simulink model "Approx_Multiplier_M3_AMA3"  (R2021a)
settings: Solver=VariableStepAuto  StartTime=0.0  StopTime=0.01  RelTol=1e-3
(part 1 of 3)
settings Model: SimulationMode=rapid-accelerator  Creator=PC  LastModifiedBy=chops

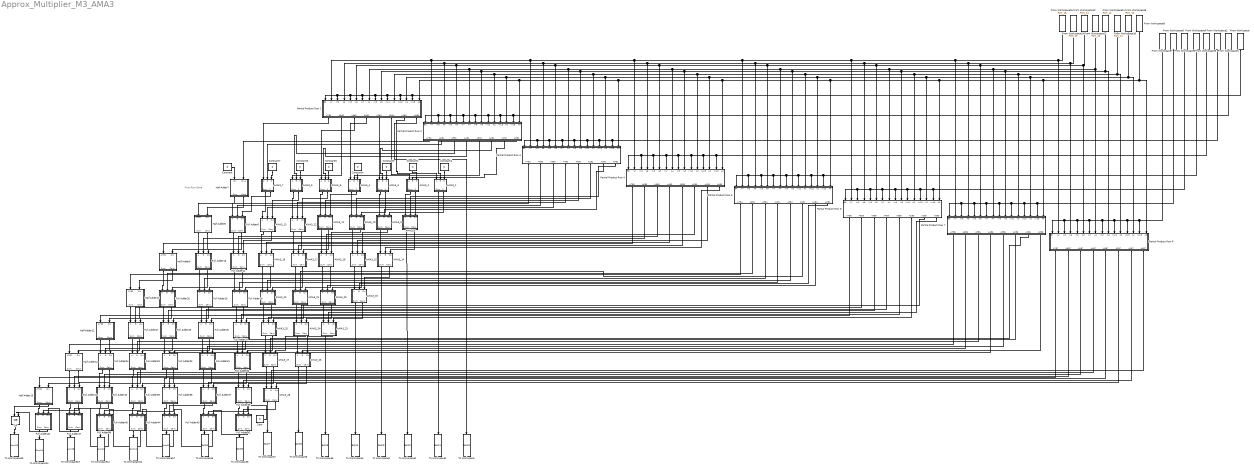
== system Approx_Multiplier_M3_AMA3 ==
  note: First Row Done
  AMA3_1 : Subsystem
  AMA3_10 : Subsystem
  AMA3_11 : Subsystem
  AMA3_12 : Subsystem
  AMA3_13 : Subsystem
  AMA3_14 : Subsystem
  AMA3_15 : Subsystem
  AMA3_16 : Subsystem
  AMA3_17 : Subsystem
  AMA3_18 : Subsystem
  AMA3_19 : Subsystem
  AMA3_2 : Subsystem
  AMA3_20 : Subsystem
  AMA3_21 : Subsystem
  AMA3_22 : Subsystem
  AMA3_23 : Subsystem
  AMA3_24 : Subsystem
  AMA3_25 : Subsystem
  AMA3_26 : Subsystem
  AMA3_27 : Subsystem
  AMA3_28 : Subsystem
  AMA3_3 : Subsystem
  AMA3_4 : Subsystem
  AMA3_5 : Subsystem
  AMA3_6 : Subsystem
  AMA3_7 : Subsystem
  AMA3_8 : Subsystem
  AMA3_9 : Subsystem
  Constant{,1..7} (8 alike) : Constant  Value=0
  From Workspace : FromWorkspace  VariableName=Port_1
  From Workspace1 : FromWorkspace  VariableName=Port_2
  From Workspace10 : FromWorkspace  VariableName=Port_11
  From Workspace11 : FromWorkspace  VariableName=Port_12
  From Workspace12 : FromWorkspace  VariableName=Port_13
  From Workspace13 : FromWorkspace  VariableName=Port_14
  From Workspace14 : FromWorkspace  VariableName=Port_15
  From Workspace15 : FromWorkspace  VariableName=Port_16
  From Workspace2 : FromWorkspace  VariableName=Port_3
  From Workspace3 : FromWorkspace  VariableName=Port_4
  From Workspace4 : FromWorkspace  VariableName=Port_5
  From Workspace5 : FromWorkspace  VariableName=Port_6
  From Workspace6 : FromWorkspace  VariableName=Port_7
  From Workspace7 : FromWorkspace  VariableName=Port_8
  From Workspace8 : FromWorkspace  VariableName=Port_9
  From Workspace9 : FromWorkspace  VariableName=Port_10
  Full Adder12 : Subsystem
  Full Adder13 : Subsystem
  Full Adder18 : Subsystem
  Full Adder19 : Subsystem
  Full Adder20 : Subsystem
  Full Adder24 : Subsystem
  Full Adder25 : Subsystem
  Full Adder26 : Subsystem
  Full Adder27 : Subsystem
  Full Adder30 : Subsystem
  Full Adder31 : Subsystem
  Full Adder32 : Subsystem
  Full Adder33 : Subsystem
  Full Adder34 : Subsystem
  Full Adder36 : Subsystem
  Full Adder37 : Subsystem
  Full Adder38 : Subsystem
  Full Adder39 : Subsystem
  Full Adder40 : Subsystem
  Full Adder41 : Subsystem
  Full Adder42 : Subsystem
  Full Adder43 : Subsystem
  Full Adder44 : Subsystem
  Full Adder45 : Subsystem
  Full Adder46 : Subsystem
  Full Adder47 : Subsystem
  Full Adder48 : Subsystem
  Full Adder6 : Subsystem
  Half Adder10 : Subsystem
  Half Adder11 : Subsystem
  Half Adder12 : Subsystem
  Half Adder13 : Subsystem
  Half Adder7 : Subsystem
  Half Adder8 : Subsystem
  Half Adder9 : Subsystem
  OR : Logic  Operator=OR  IconShape=distinctive  AllPortsSameDT=off  OutDataTypeStr=boolean
  Partial Product Row 1 : Subsystem
  Partial Product Row 2 : Subsystem
  Partial Product Row 3 : Subsystem
  Partial Product Row 4 : Subsystem
  Partial Product Row 5 : Subsystem
  Partial Product Row 6 : Subsystem
  Partial Product Row 7 : Subsystem
  Partial Product Row 8 : Subsystem
  To Workspace : ToWorkspace  VariableName=Sum0  SampleTime=0.01
      settings: Save2DSignal=2-D array (concatenate along first dimension)
  To Workspace1 : ToWorkspace  VariableName=Sum1  SampleTime=0.01
      settings: Save2DSignal=2-D array (concatenate along first dimension)
  To Workspace10 : ToWorkspace  VariableName=Sum10  SampleTime=0.01
      settings: Save2DSignal=2-D array (concatenate along first dimension)
  To Workspace11 : ToWorkspace  VariableName=Sum11  SampleTime=0.01
      settings: Save2DSignal=2-D array (concatenate along first dimension)
  To Workspace12 : ToWorkspace  VariableName=Sum12  SampleTime=0.01
      settings: Save2DSignal=2-D array (concatenate along first dimension)
  To Workspace13 : ToWorkspace  VariableName=Sum13  SampleTime=0.01
      settings: Save2DSignal=2-D array (concatenate along first dimension)
  To Workspace14 : ToWorkspace  VariableName=Sum14  SampleTime=0.01
      settings: Save2DSignal=2-D array (concatenate along first dimension)
  To Workspace15 : ToWorkspace  VariableName=Sum15  SampleTime=0.01
      settings: Save2DSignal=2-D array (concatenate along first dimension)
  To Workspace2 : ToWorkspace  VariableName=Sum2  SampleTime=0.01
      settings: Save2DSignal=2-D array (concatenate along first dimension)
  To Workspace3 : ToWorkspace  VariableName=Sum3  SampleTime=0.01
      settings: Save2DSignal=2-D array (concatenate along first dimension)
  To Workspace4 : ToWorkspace  VariableName=Sum4  SampleTime=0.01
      settings: Save2DSignal=2-D array (concatenate along first dimension)
  To Workspace5 : ToWorkspace  VariableName=Sum5  SampleTime=0.01
      settings: Save2DSignal=2-D array (concatenate along first dimension)
  To Workspace6 : ToWorkspace  VariableName=Sum6  SampleTime=0.01
      settings: Save2DSignal=2-D array (concatenate along first dimension)
  To Workspace7 : ToWorkspace  VariableName=Sum7  SampleTime=0.01
      settings: Save2DSignal=2-D array (concatenate along first dimension)
  To Workspace8 : ToWorkspace  VariableName=Sum8  SampleTime=0.01
      settings: Save2DSignal=2-D array (concatenate along first dimension)
  To Workspace9 : ToWorkspace  VariableName=Sum9  SampleTime=0.01
      settings: Save2DSignal=2-D array (concatenate along first dimension)
  Zero : Constant  Value=0  OutDataTypeStr=Inherit: Inherit via back propagation
  wires:
  Half Adder11/2(Cout) -> Half Adder12/2(Cin)
  AMA3_8/1(Sum) -> To Workspace2/1
  AMA3_12/2(Carry) -> AMA3_18/3(Cin)
  Full Adder46/1(Sum) -> To Workspace12/1
  Partial Product Row 1/5(A3B0) -> AMA3_3/1(A)
  Full Adder43/1(Sum) -> To Workspace9/1
  From Workspace13/1 -> Partial Product Row 8/6(A5), Partial Product Row 6/6(A5), Partial Product Row 3/6(A5), Partial Product Row 1/6(A5), Partial Product Row 2/6(A5), Partial Product Row 4/6(A5), Partial Product Row 5/6(A5), Partial Product Row 7/6(A5)
  AMA3_9/2(Carry) -> AMA3_15/3(Cin)
  Partial Product Row 2/5(A3B1) -> AMA3_4/2(B)
  Partial Product Row 7/2(A6B6) -> Full Adder34/2(B)
  Partial Product Row 1/4(A4B0) -> AMA3_4/1(A)
  Partial Product Row 8/6(A2B7) -> Full Adder37/2(B)
  Partial Product Row 8/3(A5B7) -> Full Adder40/2(B)
  AMA3_10/2(Carry) -> AMA3_16/3(Cin)
  Partial Product Row 6/8(A0B5) -> AMA3_23/2(B)
  AMA3_7/1(Sum) -> AMA3_13/1(A)
  Full Adder47/1(Sum) -> To Workspace13/1
  AMA3_9/1(Sum) -> AMA3_14/1(A)
  AMA3_5/1(Sum) -> AMA3_11/1(A)
  From Workspace7/1 -> Partial Product Row 8/11(In11), Partial Product Row 8/9(In9), Partial Product Row 8/7(In7), Partial Product Row 8/5(In5), Partial Product Row 8/3(In3), Partial Product Row 8/1(B7), Partial Product Row 8/13(In13), Partial Product Row 8/15(In15)
  AMA3_10/1(Sum) -> AMA3_15/1(A)
  Partial Product Row 4/6(A2B3) -> AMA3_16/2(B)
  Partial Product Row 3/5(A3B2) -> AMA3_11/2(B)
  Half Adder10/1(Sum) -> Full Adder27/1(A)
  AMA3_21/2(Carry) -> AMA3_25/3(Cin)
  Partial Product Row 1/8(A0B0) -> To Workspace/1
  AMA3_17/2(Carry) -> AMA3_22/3(Cin)
  Partial Product Row 7/8(A0B6) -> AMA3_26/2(B)
  Half Adder12/2(Cout) -> Half Adder13/2(Cin)
  AMA3_19/1(Sum) -> To Workspace4/1
  AMA3_21/1(Sum) -> AMA3_24/1(A)
  Full Adder43/2(Carry) -> Full Adder44/3(Cin)
  Full Adder20/2(Carry) -> Full Adder27/3(Cin)
  Partial Product Row 6/1(A7B5) -> Half Adder11/1(A7B2)
  Full Adder31/2(Carry) -> Full Adder38/3(Cin)
  Partial Product Row 3/3(A5B2) -> AMA3_13/2(B)
  From Workspace5/1 -> Partial Product Row 6/7(In7), Partial Product Row 6/5(In5), Partial Product Row 6/1(B5), Partial Product Row 6/3(In3), Partial Product Row 6/9(In9), Partial Product Row 6/11(In11), Partial Product Row 6/13(In13), Partial Product Row 6/15(In15)
  AMA3_23/1(Sum) -> To Workspace5/1
  Partial Product Row 3/6(A2B2) -> AMA3_10/2(B)
  AMA3_4/1(Sum) -> AMA3_10/1(A)
  From Workspace11/1 -> Partial Product Row 8/10(A3), Partial Product Row 6/10(A3), Partial Product Row 4/10(A3), Partial Product Row 3/10(A3), Partial Product Row 1/10(A3), Partial Product Row 2/10(A3), Partial Product Row 5/10(A3), Partial Product Row 7/10(A3)
  Full Adder26/2(Carry) -> Full Adder33/3(Cin)
  From Workspace15/1 -> Partial Product Row 7/2(A7), Partial Product Row 5/2(A7), Partial Product Row 3/2(A7), Partial Product Row 1/2(A7), Partial Product Row 2/2(A7), Partial Product Row 4/2(A7), Partial Product Row 6/2(A7), Partial Product Row 8/2(A7)
  Partial Product Row 7/4(A4B6) -> Full Adder32/2(B)
  Full Adder31/1(Sum) -> Full Adder37/1(A)
  Full Adder24/2(Carry) -> Full Adder31/3(Cin)
  Full Adder34/1(Sum) -> Full Adder40/1(A)
  Full Adder30/1(Sum) -> Full Adder36/1(A)
  Partial Product Row 6/2(A6B5) -> Full Adder27/2(B)
  Full Adder41/1(Sum) -> Full Adder47/1(A)
  Partial Product Row 2/2(A6B1) -> AMA3_7/2(B)
  Partial Product Row 8/7(A1B7) -> Full Adder36/2(B)
  From Workspace8/1 -> Partial Product Row 8/16(A0), Partial Product Row 7/16(A0), Partial Product Row 6/16(A0), Partial Product Row 4/16(A0), Partial Product Row 3/16(A0), Partial Product Row 1/16(A0), Partial Product Row 2/16(A0), Partial Product Row 5/16(A0)
  AMA3_15/1(Sum) -> AMA3_19/1(A)
  Half Adder7/1(Sum) -> Full Adder6/1(A)
  Constant/1 -> Half Adder7/1(Cin)
  AMA3_4/2(Carry) -> AMA3_11/3(Cin)
  AMA3_18/1(Sum) -> AMA3_22/1(A)
  Constant7/1 -> AMA3_7/3(Cin)
  Full Adder19/1(Sum) -> Full Adder25/1(A)
  Constant5/1 -> AMA3_5/3(Cin)
  AMA3_27/2(Carry) -> Full Adder36/3(Cin)
  Partial Product Row 6/3(A5B5) -> Full Adder26/2(B)
  Partial Product Row 2/1(A7B1) -> Half Adder7/2(Cin1)
  AMA3_2/1(Sum) -> AMA3_8/1(A)
  Partial Product Row 5/5(A3B4) -> AMA3_22/2(B)
  AMA3_20/2(Carry) -> AMA3_24/3(Cin)
  Partial Product Row 8/2(A6B7) -> Full Adder41/2(B)
  From Workspace2/1 -> Partial Product Row 3/13(In13), Partial Product Row 3/7(In7), Partial Product Row 3/5(In5), Partial Product Row 3/3(In3), Partial Product Row 3/1(B2), Partial Product Row 3/9(In9), Partial Product Row 3/11(In11), Partial Product Row 3/15(In15)
  Partial Product Row 2/8(A0B1) -> AMA3_1/2(B)
  Constant1/1 -> AMA3_1/3(Cin)
  Partial Product Row 3/4(A4B2) -> AMA3_12/2(B)
  Partial Product Row 5/2(A6B4) -> Full Adder20/2(B)
  Full Adder27/1(Sum) -> Full Adder33/1(A)
  AMA3_12/1(Sum) -> AMA3_17/1(A)
  AMA3_26/1(Sum) -> To Workspace6/1
  From Workspace10/1 -> Partial Product Row 8/12(A2), Partial Product Row 7/12(A2), Partial Product Row 5/12(A2), Partial Product Row 4/12(A2), Partial Product Row 3/12(A2), Partial Product Row 1/12(A2), Partial Product Row 2/12(A2), Partial Product Row 6/12(A2)
  Full Adder40/1(Sum) -> Full Adder46/1(A)
  Partial Product Row 6/5(A3B5) -> Full Adder24/2(B)
  AMA3_28/1(Sum) -> To Workspace7/1
  Partial Product Row 1/3(A5B0) -> AMA3_5/1(A)
  Constant6/1 -> AMA3_6/3(Cin)
  Half Adder8/1(Sum) -> Full Adder13/1(A)
  AMA3_17/1(Sum) -> AMA3_21/1(A)
  Partial Product Row 8/5(A3B7) -> Full Adder38/2(B)
  From Workspace1/1 -> Partial Product Row 2/15(In15), Partial Product Row 2/5(In5), Partial Product Row 2/3(In3), Partial Product Row 2/1(B1), Partial Product Row 2/7(In7), Partial Product Row 2/9(In9), Partial Product Row 2/11(In11), Partial Product Row 2/13(In13)
  AMA3_16/1(Sum) -> AMA3_20/1(A)
  Partial Product Row 7/1(A7B6) -> Half Adder12/1(A7B2)
  Partial Product Row 7/7(A1B6) -> AMA3_27/2(B)
  AMA3_15/2(Carry) -> AMA3_20/3(Cin)
  Partial Product Row 4/2(A6B3) -> Full Adder13/2(B)
  AMA3_2/2(Carry) -> AMA3_9/3(Cin)
  AMA3_3/1(Sum) -> AMA3_9/1(A)
  Full Adder42/2(Carry) -> Full Adder43/3(Cin)
  AMA3_24/2(Carry) -> AMA3_27/3(Cin)
  AMA3_13/1(Sum) -> AMA3_18/1(A)
  Full Adder32/1(Sum) -> Full Adder38/1(A)
  Full Adder37/1(Sum) -> Full Adder43/1(A)
  Partial Product Row 8/4(A4B7) -> Full Adder39/2(B)
  AMA3_1/1(Sum) -> To Workspace1/1
  AMA3_3/2(Carry) -> AMA3_10/3(Cin)
  Partial Product Row 1/6(A2B0) -> AMA3_2/1(A)
  Half Adder8/2(Cout) -> Half Adder9/2(Cin)
  Partial Product Row 4/4(A4B3) -> AMA3_18/2(B)
  Partial Product Row 6/6(A2B5) -> AMA3_25/2(B)
  Partial Product Row 5/3(A5B4) -> Full Adder19/2(B)
  From Workspace3/1 -> Partial Product Row 4/13(In13), Partial Product Row 4/11(In11), Partial Product Row 4/9(In9), Partial Product Row 4/5(In5), Partial Product Row 4/3(In3), Partial Product Row 4/1(B3), Partial Product Row 4/7(In7), Partial Product Row 4/15(In15)
  Full Adder12/2(Carry) -> Full Adder19/3(Cin)
  From Workspace6/1 -> Partial Product Row 7/13(In13), Partial Product Row 7/7(In7), Partial Product Row 7/5(In5), Partial Product Row 7/1(B6), Partial Product Row 7/3(In3), Partial Product Row 7/9(In9), Partial Product Row 7/11(In11), Partial Product Row 7/15(In15)
  Full Adder30/2(Carry) -> Full Adder37/3(Cin)
  AMA3_23/2(Carry) -> AMA3_26/3(Cin)
  Full Adder44/1(Sum) -> To Workspace10/1
  AMA3_6/2(Carry) -> AMA3_13/3(Cin)
  AMA3_16/2(Carry) -> AMA3_21/3(Cin)
  From Workspace14/1 -> Partial Product Row 8/4(A6), Partial Product Row 7/4(A6), Partial Product Row 6/4(A6), Partial Product Row 5/4(A6), Partial Product Row 4/4(A6), Partial Product Row 3/4(A6), Partial Product Row 1/4(A6), Partial Product Row 2/4(A6)
  Partial Product Row 5/7(A1B4) -> AMA3_20/2(B)
  Half Adder12/1(Sum) -> Full Adder41/1(A)
  Full Adder12/1(Sum) -> Full Adder18/1(A)
  Partial Product Row 4/1(A7B3) -> Half Adder9/1(A7B2)
  From Workspace4/1 -> Partial Product Row 5/15(In15), Partial Product Row 5/13(In13), Partial Product Row 5/11(In11), Partial Product Row 5/7(In7), Partial Product Row 5/5(In5), Partial Product Row 5/1(B4), Partial Product Row 5/3(In3), Partial Product Row 5/9(In9)
  Full Adder25/1(Sum) -> Full Adder31/1(A)
  AMA3_7/2(Carry) -> Full Adder6/3(Cin)
  Half Adder13/1(Sum) -> Full Adder48/1(A)
  Full Adder33/1(Sum) -> Full Adder39/1(A)
  From Workspace9/1 -> Partial Product Row 8/14(A1), Partial Product Row 7/14(A1), Partial Product Row 4/14(A1), Partial Product Row 1/14(A1), Partial Product Row 2/14(A1), Partial Product Row 3/14(A1), Partial Product Row 5/14(A1), Partial Product Row 6/14(A1)
  AMA3_14/1(Sum) -> To Workspace3/1
  AMA3_20/1(Sum) -> AMA3_23/1(A)
  Partial Product Row 1/1(A7B0) -> AMA3_7/1(A)
  Partial Product Row 7/3(A5B6) -> Full Adder33/2(B)
  Full Adder18/1(Sum) -> Full Adder24/1(A)
  From Workspace12/1 -> Partial Product Row 8/8(A4), Partial Product Row 6/8(A4), Partial Product Row 4/8(A4), Partial Product Row 3/8(A4), Partial Product Row 1/8(A4), Partial Product Row 2/8(A4), Partial Product Row 5/8(A4), Partial Product Row 7/8(A4)
  AMA3_11/2(Carry) -> AMA3_17/3(Cin)
  AMA3_19/2(Carry) -> AMA3_23/3(Cin)
  Full Adder26/1(Sum) -> Full Adder32/1(A)
  Partial Product Row 1/7(A1B0) -> AMA3_1/1(A)
  Full Adder46/2(Carry) -> Full Adder47/3(Cin)
  Partial Product Row 4/7(A1B3) -> AMA3_15/2(B)
  Partial Product Row 5/1(A7B4) -> Half Adder10/1(A7B2)
  Full Adder33/2(Carry) -> Full Adder40/3(Cin)
  Half Adder9/1(Sum) -> Full Adder20/1(A)
  Partial Product Row 4/3(A5B3) -> Full Adder12/2(B)
  Full Adder27/2(Carry) -> Full Adder34/3(Cin)
  Full Adder34/2(Carry) -> Full Adder41/3(Cin)
  Full Adder20/1(Sum) -> Full Adder26/1(A)
  Partial Product Row 8/8(A0B7) -> AMA3_28/2(B)
  AMA3_6/1(Sum) -> AMA3_12/1(A)
  Full Adder36/1(Sum) -> Full Adder42/1(A)
  Partial Product Row 2/7(A1B1) -> AMA3_2/2(B)
  Partial Product Row 5/6(A2B4) -> AMA3_21/2(B)
  Full Adder6/1(Sum) -> Full Adder12/1(A)
  Full Adder45/2(Carry) -> Full Adder46/3(Cin)
  AMA3_11/1(Sum) -> AMA3_16/1(A)
  AMA3_13/2(Carry) -> Full Adder12/3(Cin)
  Partial Product Row 2/4(A4B1) -> AMA3_5/2(B)
  Partial Product Row 4/8(A0B3) -> AMA3_14/2(B)
  Partial Product Row 2/3(A5B1) -> AMA3_6/2(B)
  Partial Product Row 6/4(A4B5) -> Full Adder25/2(B)
  AMA3_1/2(Carry) -> AMA3_8/3(Cin)
  Full Adder48/1(Sum) -> To Workspace14/1
  From Workspace/1 -> Partial Product Row 1/3(In3), Partial Product Row 1/1(B0), Partial Product Row 1/5(In5), Partial Product Row 1/7(In7), Partial Product Row 1/9(In9), Partial Product Row 1/11(In11), Partial Product Row 1/13(In13), Partial Product Row 1/15(In15)
  AMA3_8/2(Carry) -> AMA3_14/3(Cin)
  Half Adder10/2(Cout) -> Half Adder11/2(Cin)
  Partial Product Row 3/8(A0B2) -> AMA3_8/2(B)
  AMA3_18/2(Carry) -> Full Adder18/3(Cin)
  Full Adder13/2(Carry) -> Full Adder20/3(Cin)
  Partial Product Row 7/6(A2B6) -> Full Adder30/2(B)
  Constant3/1 -> AMA3_3/3(Cin)
  AMA3_27/1(Sum) -> AMA3_28/1(A)
  AMA3_25/2(Carry) -> Full Adder30/3(Cin)
  Full Adder25/2(Carry) -> Full Adder32/3(Cin)
  Partial Product Row 4/5(A3B3) -> AMA3_17/2(B)
  AMA3_25/1(Sum) -> AMA3_27/1(A)
  Full Adder42/1(Sum) -> To Workspace8/1
  Half Adder11/1(Sum) -> Full Adder34/1(A)
  AMA3_5/2(Carry) -> AMA3_12/3(Cin)
  Partial Product Row 6/7(A1B5) -> AMA3_24/2(B)
  Constant4/1 -> AMA3_4/3(Cin)
  Constant2/1 -> AMA3_2/3(Cin)
  Full Adder47/2(Carry) -> Full Adder48/3(Cin)
  Full Adder39/1(Sum) -> Full Adder45/1(A)
  Full Adder18/2(Carry) -> Full Adder25/3(Cin)
  Partial Product Row 7/5(A3B6) -> Full Adder31/2(B)
  Partial Product Row 5/4(A4B4) -> Full Adder18/2(B)
  Half Adder9/2(Cout) -> Half Adder10/2(Cin)
  Partial Product Row 3/1(A7B2) -> Half Adder8/1(A7B2)
  Half Adder7/2(Cout) -> Half Adder8/2(Cin)
  Partial Product Row 3/2(A6B2) -> Full Adder6/2(B)
  Partial Product Row 5/8(A0B4) -> AMA3_19/2(B)
  AMA3_22/1(Sum) -> AMA3_25/1(A)
  Partial Product Row 3/7(A1B2) -> AMA3_9/2(B)
  Full Adder44/2(Carry) -> Full Adder45/3(Cin)
  Partial Product Row 1/2(A6B0) -> AMA3_6/1(A)
  Partial Product Row 2/6(A2B1) -> AMA3_3/2(B)
  Full Adder6/2(Carry) -> Full Adder13/3(Cin)
  AMA3_14/2(Carry) -> AMA3_19/3(Cin)
  Partial Product Row 8/1(A7B7) -> Half Adder13/1(A7B2)
  Full Adder24/1(Sum) -> Full Adder30/1(A)
  Full Adder13/1(Sum) -> Full Adder19/1(A)
  Full Adder38/1(Sum) -> Full Adder44/1(A)
  Full Adder45/1(Sum) -> To Workspace11/1
  Full Adder32/2(Carry) -> Full Adder39/3(Cin)
  AMA3_22/2(Carry) -> Full Adder24/3(Cin)
  AMA3_24/1(Sum) -> AMA3_26/1(A)
  Full Adder19/2(Carry) -> Full Adder26/3(Cin)
  AMA3_26/2(Carry) -> AMA3_28/3(Cin)
  Full Adder48/2(Carry) -> OR/2
  Half Adder13/2(Cout) -> OR/1
  OR/1 -> To Workspace15/1
  AMA3_28/2(Carry) -> Full Adder42/2(B)
  Full Adder36/2(Carry) -> Full Adder43/2(B)
  Full Adder37/2(Carry) -> Full Adder44/2(B)
  Full Adder38/2(Carry) -> Full Adder45/2(B)
  Full Adder39/2(Carry) -> Full Adder46/2(B)
  Full Adder40/2(Carry) -> Full Adder47/2(B)
  Full Adder41/2(Carry) -> Full Adder48/2(B)
  Zero/1 -> Full Adder42/3(Cin)

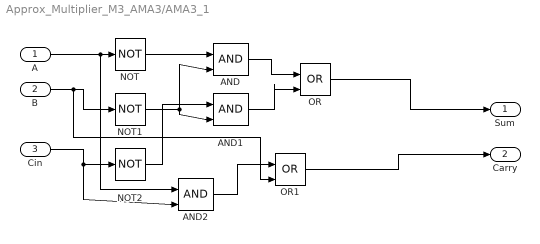
== system Approx_Multiplier_M3_AMA3/AMA3_1 ==
  A : Inport
  B : Inport  Port=2
  Cin : Inport  Port=3
  AND : Logic  IconShape=distinctive  AllPortsSameDT=off  OutDataTypeStr=boolean
  AND1 : Logic  IconShape=distinctive  AllPortsSameDT=off  OutDataTypeStr=boolean
  AND2 : Logic  IconShape=distinctive  AllPortsSameDT=off  OutDataTypeStr=boolean
  NOT : Logic  Operator=NOT  IconShape=distinctive  AllPortsSameDT=off  OutDataTypeStr=boolean
  NOT1 : Logic  Operator=NOT  IconShape=distinctive  AllPortsSameDT=off  OutDataTypeStr=boolean
  NOT2 : Logic  Operator=NOT  IconShape=distinctive  AllPortsSameDT=off  OutDataTypeStr=boolean
  OR : Logic  Operator=OR  IconShape=distinctive  AllPortsSameDT=off  OutDataTypeStr=boolean
  OR1 : Logic  Operator=OR  IconShape=distinctive  AllPortsSameDT=off  OutDataTypeStr=boolean
  Sum : Outport
  Carry : Outport  Port=2
  wires:
  A/1 -> AND2/1, NOT/1
  B/1 -> OR1/2, NOT1/1
  NOT/1 -> AND/1
  NOT1/1 -> AND1/2, AND/2
  Cin/1 -> AND2/2, NOT2/1
  NOT2/1 -> AND1/1
  AND/1 -> OR/1
  AND1/1 -> OR/2
  OR/1 -> Sum/1
  AND2/1 -> OR1/1
  OR1/1 -> Carry/1

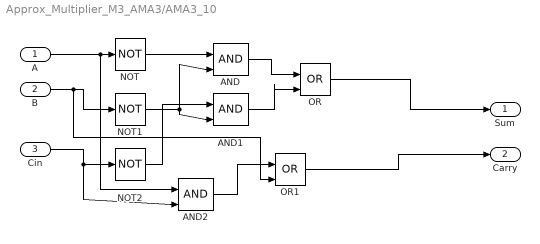
== system Approx_Multiplier_M3_AMA3/AMA3_10 ==
  A : Inport
  B : Inport  Port=2
  Cin : Inport  Port=3
  AND : Logic  IconShape=distinctive  AllPortsSameDT=off  OutDataTypeStr=boolean
  AND1 : Logic  IconShape=distinctive  AllPortsSameDT=off  OutDataTypeStr=boolean
  AND2 : Logic  IconShape=distinctive  AllPortsSameDT=off  OutDataTypeStr=boolean
  NOT : Logic  Operator=NOT  IconShape=distinctive  AllPortsSameDT=off  OutDataTypeStr=boolean
  NOT1 : Logic  Operator=NOT  IconShape=distinctive  AllPortsSameDT=off  OutDataTypeStr=boolean
  NOT2 : Logic  Operator=NOT  IconShape=distinctive  AllPortsSameDT=off  OutDataTypeStr=boolean
  OR : Logic  Operator=OR  IconShape=distinctive  AllPortsSameDT=off  OutDataTypeStr=boolean
  OR1 : Logic  Operator=OR  IconShape=distinctive  AllPortsSameDT=off  OutDataTypeStr=boolean
  Sum : Outport
  Carry : Outport  Port=2
  wires:
  A/1 -> AND2/1, NOT/1
  B/1 -> OR1/2, NOT1/1
  NOT/1 -> AND/1
  NOT1/1 -> AND1/2, AND/2
  Cin/1 -> AND2/2, NOT2/1
  NOT2/1 -> AND1/1
  AND/1 -> OR/1
  AND1/1 -> OR/2
  OR/1 -> Sum/1
  AND2/1 -> OR1/1
  OR1/1 -> Carry/1

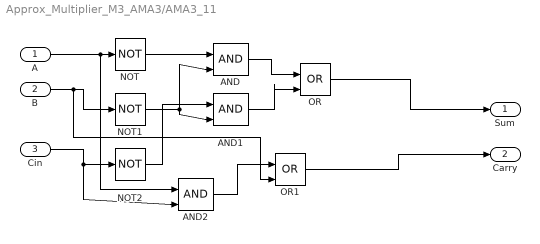
== system Approx_Multiplier_M3_AMA3/AMA3_11 ==
  A : Inport
  B : Inport  Port=2
  Cin : Inport  Port=3
  AND : Logic  IconShape=distinctive  AllPortsSameDT=off  OutDataTypeStr=boolean
  AND1 : Logic  IconShape=distinctive  AllPortsSameDT=off  OutDataTypeStr=boolean
  AND2 : Logic  IconShape=distinctive  AllPortsSameDT=off  OutDataTypeStr=boolean
  NOT : Logic  Operator=NOT  IconShape=distinctive  AllPortsSameDT=off  OutDataTypeStr=boolean
  NOT1 : Logic  Operator=NOT  IconShape=distinctive  AllPortsSameDT=off  OutDataTypeStr=boolean
  NOT2 : Logic  Operator=NOT  IconShape=distinctive  AllPortsSameDT=off  OutDataTypeStr=boolean
  OR : Logic  Operator=OR  IconShape=distinctive  AllPortsSameDT=off  OutDataTypeStr=boolean
  OR1 : Logic  Operator=OR  IconShape=distinctive  AllPortsSameDT=off  OutDataTypeStr=boolean
  Sum : Outport
  Carry : Outport  Port=2
  wires:
  A/1 -> AND2/1, NOT/1
  B/1 -> OR1/2, NOT1/1
  NOT/1 -> AND/1
  NOT1/1 -> AND1/2, AND/2
  Cin/1 -> AND2/2, NOT2/1
  NOT2/1 -> AND1/1
  AND/1 -> OR/1
  AND1/1 -> OR/2
  OR/1 -> Sum/1
  AND2/1 -> OR1/1
  OR1/1 -> Carry/1

== system Approx_Multiplier_M3_AMA3/AMA3_12 ==
  A : Inport
  B : Inport  Port=2
  Cin : Inport  Port=3
  AND : Logic  IconShape=distinctive  AllPortsSameDT=off  OutDataTypeStr=boolean
  AND1 : Logic  IconShape=distinctive  AllPortsSameDT=off  OutDataTypeStr=boolean
  AND2 : Logic  IconShape=distinctive  AllPortsSameDT=off  OutDataTypeStr=boolean
  NOT : Logic  Operator=NOT  IconShape=distinctive  AllPortsSameDT=off  OutDataTypeStr=boolean
  NOT1 : Logic  Operator=NOT  IconShape=distinctive  AllPortsSameDT=off  OutDataTypeStr=boolean
  NOT2 : Logic  Operator=NOT  IconShape=distinctive  AllPortsSameDT=off  OutDataTypeStr=boolean
  OR : Logic  Operator=OR  IconShape=distinctive  AllPortsSameDT=off  OutDataTypeStr=boolean
  OR1 : Logic  Operator=OR  IconShape=distinctive  AllPortsSameDT=off  OutDataTypeStr=boolean
  Sum : Outport
  Carry : Outport  Port=2
  wires:
  A/1 -> AND2/1, NOT/1
  B/1 -> OR1/2, NOT1/1
  NOT/1 -> AND/1
  NOT1/1 -> AND1/2, AND/2
  Cin/1 -> AND2/2, NOT2/1
  NOT2/1 -> AND1/1
  AND/1 -> OR/1
  AND1/1 -> OR/2
  OR/1 -> Sum/1
  AND2/1 -> OR1/1
  OR1/1 -> Carry/1

== system Approx_Multiplier_M3_AMA3/AMA3_13 ==
  A : Inport
  B : Inport  Port=2
  Cin : Inport  Port=3
  AND : Logic  IconShape=distinctive  AllPortsSameDT=off  OutDataTypeStr=boolean
  AND1 : Logic  IconShape=distinctive  AllPortsSameDT=off  OutDataTypeStr=boolean
  AND2 : Logic  IconShape=distinctive  AllPortsSameDT=off  OutDataTypeStr=boolean
  NOT : Logic  Operator=NOT  IconShape=distinctive  AllPortsSameDT=off  OutDataTypeStr=boolean
  NOT1 : Logic  Operator=NOT  IconShape=distinctive  AllPortsSameDT=off  OutDataTypeStr=boolean
  NOT2 : Logic  Operator=NOT  IconShape=distinctive  AllPortsSameDT=off  OutDataTypeStr=boolean
  OR : Logic  Operator=OR  IconShape=distinctive  AllPortsSameDT=off  OutDataTypeStr=boolean
  OR1 : Logic  Operator=OR  IconShape=distinctive  AllPortsSameDT=off  OutDataTypeStr=boolean
  Sum : Outport
  Carry : Outport  Port=2
  wires:
  A/1 -> AND2/1, NOT/1
  B/1 -> OR1/2, NOT1/1
  NOT/1 -> AND/1
  NOT1/1 -> AND1/2, AND/2
  Cin/1 -> AND2/2, NOT2/1
  NOT2/1 -> AND1/1
  AND/1 -> OR/1
  AND1/1 -> OR/2
  OR/1 -> Sum/1
  AND2/1 -> OR1/1
  OR1/1 -> Carry/1

== system Approx_Multiplier_M3_AMA3/AMA3_14 ==
  A : Inport
  B : Inport  Port=2
  Cin : Inport  Port=3
  AND : Logic  IconShape=distinctive  AllPortsSameDT=off  OutDataTypeStr=boolean
  AND1 : Logic  IconShape=distinctive  AllPortsSameDT=off  OutDataTypeStr=boolean
  AND2 : Logic  IconShape=distinctive  AllPortsSameDT=off  OutDataTypeStr=boolean
  NOT : Logic  Operator=NOT  IconShape=distinctive  AllPortsSameDT=off  OutDataTypeStr=boolean
  NOT1 : Logic  Operator=NOT  IconShape=distinctive  AllPortsSameDT=off  OutDataTypeStr=boolean
  NOT2 : Logic  Operator=NOT  IconShape=distinctive  AllPortsSameDT=off  OutDataTypeStr=boolean
  OR : Logic  Operator=OR  IconShape=distinctive  AllPortsSameDT=off  OutDataTypeStr=boolean
  OR1 : Logic  Operator=OR  IconShape=distinctive  AllPortsSameDT=off  OutDataTypeStr=boolean
  Sum : Outport
  Carry : Outport  Port=2
  wires:
  A/1 -> AND2/1, NOT/1
  B/1 -> OR1/2, NOT1/1
  NOT/1 -> AND/1
  NOT1/1 -> AND1/2, AND/2
  Cin/1 -> AND2/2, NOT2/1
  NOT2/1 -> AND1/1
  AND/1 -> OR/1
  AND1/1 -> OR/2
  OR/1 -> Sum/1
  AND2/1 -> OR1/1
  OR1/1 -> Carry/1

== system Approx_Multiplier_M3_AMA3/AMA3_15 ==
  A : Inport
  B : Inport  Port=2
  Cin : Inport  Port=3
  AND : Logic  IconShape=distinctive  AllPortsSameDT=off  OutDataTypeStr=boolean
  AND1 : Logic  IconShape=distinctive  AllPortsSameDT=off  OutDataTypeStr=boolean
  AND2 : Logic  IconShape=distinctive  AllPortsSameDT=off  OutDataTypeStr=boolean
  NOT : Logic  Operator=NOT  IconShape=distinctive  AllPortsSameDT=off  OutDataTypeStr=boolean
  NOT1 : Logic  Operator=NOT  IconShape=distinctive  AllPortsSameDT=off  OutDataTypeStr=boolean
  NOT2 : Logic  Operator=NOT  IconShape=distinctive  AllPortsSameDT=off  OutDataTypeStr=boolean
  OR : Logic  Operator=OR  IconShape=distinctive  AllPortsSameDT=off  OutDataTypeStr=boolean
  OR1 : Logic  Operator=OR  IconShape=distinctive  AllPortsSameDT=off  OutDataTypeStr=boolean
  Sum : Outport
  Carry : Outport  Port=2
  wires:
  A/1 -> AND2/1, NOT/1
  B/1 -> OR1/2, NOT1/1
  NOT/1 -> AND/1
  NOT1/1 -> AND1/2, AND/2
  Cin/1 -> AND2/2, NOT2/1
  NOT2/1 -> AND1/1
  AND/1 -> OR/1
  AND1/1 -> OR/2
  OR/1 -> Sum/1
  AND2/1 -> OR1/1
  OR1/1 -> Carry/1

== system Approx_Multiplier_M3_AMA3/AMA3_16 ==
  A : Inport
  B : Inport  Port=2
  Cin : Inport  Port=3
  AND : Logic  IconShape=distinctive  AllPortsSameDT=off  OutDataTypeStr=boolean
  AND1 : Logic  IconShape=distinctive  AllPortsSameDT=off  OutDataTypeStr=boolean
  AND2 : Logic  IconShape=distinctive  AllPortsSameDT=off  OutDataTypeStr=boolean
  NOT : Logic  Operator=NOT  IconShape=distinctive  AllPortsSameDT=off  OutDataTypeStr=boolean
  NOT1 : Logic  Operator=NOT  IconShape=distinctive  AllPortsSameDT=off  OutDataTypeStr=boolean
  NOT2 : Logic  Operator=NOT  IconShape=distinctive  AllPortsSameDT=off  OutDataTypeStr=boolean
  OR : Logic  Operator=OR  IconShape=distinctive  AllPortsSameDT=off  OutDataTypeStr=boolean
  OR1 : Logic  Operator=OR  IconShape=distinctive  AllPortsSameDT=off  OutDataTypeStr=boolean
  Sum : Outport
  Carry : Outport  Port=2
  wires:
  A/1 -> AND2/1, NOT/1
  B/1 -> OR1/2, NOT1/1
  NOT/1 -> AND/1
  NOT1/1 -> AND1/2, AND/2
  Cin/1 -> AND2/2, NOT2/1
  NOT2/1 -> AND1/1
  AND/1 -> OR/1
  AND1/1 -> OR/2
  OR/1 -> Sum/1
  AND2/1 -> OR1/1
  OR1/1 -> Carry/1

== system Approx_Multiplier_M3_AMA3/AMA3_17 ==
  A : Inport
  B : Inport  Port=2
  Cin : Inport  Port=3
  AND : Logic  IconShape=distinctive  AllPortsSameDT=off  OutDataTypeStr=boolean
  AND1 : Logic  IconShape=distinctive  AllPortsSameDT=off  OutDataTypeStr=boolean
  AND2 : Logic  IconShape=distinctive  AllPortsSameDT=off  OutDataTypeStr=boolean
  NOT : Logic  Operator=NOT  IconShape=distinctive  AllPortsSameDT=off  OutDataTypeStr=boolean
  NOT1 : Logic  Operator=NOT  IconShape=distinctive  AllPortsSameDT=off  OutDataTypeStr=boolean
  NOT2 : Logic  Operator=NOT  IconShape=distinctive  AllPortsSameDT=off  OutDataTypeStr=boolean
  OR : Logic  Operator=OR  IconShape=distinctive  AllPortsSameDT=off  OutDataTypeStr=boolean
  OR1 : Logic  Operator=OR  IconShape=distinctive  AllPortsSameDT=off  OutDataTypeStr=boolean
  Sum : Outport
  Carry : Outport  Port=2
  wires:
  A/1 -> AND2/1, NOT/1
  B/1 -> OR1/2, NOT1/1
  NOT/1 -> AND/1
  NOT1/1 -> AND1/2, AND/2
  Cin/1 -> AND2/2, NOT2/1
  NOT2/1 -> AND1/1
  AND/1 -> OR/1
  AND1/1 -> OR/2
  OR/1 -> Sum/1
  AND2/1 -> OR1/1
  OR1/1 -> Carry/1

== system Approx_Multiplier_M3_AMA3/AMA3_18 ==
  A : Inport
  B : Inport  Port=2
  Cin : Inport  Port=3
  AND : Logic  IconShape=distinctive  AllPortsSameDT=off  OutDataTypeStr=boolean
  AND1 : Logic  IconShape=distinctive  AllPortsSameDT=off  OutDataTypeStr=boolean
  AND2 : Logic  IconShape=distinctive  AllPortsSameDT=off  OutDataTypeStr=boolean
  NOT : Logic  Operator=NOT  IconShape=distinctive  AllPortsSameDT=off  OutDataTypeStr=boolean
  NOT1 : Logic  Operator=NOT  IconShape=distinctive  AllPortsSameDT=off  OutDataTypeStr=boolean
  NOT2 : Logic  Operator=NOT  IconShape=distinctive  AllPortsSameDT=off  OutDataTypeStr=boolean
  OR : Logic  Operator=OR  IconShape=distinctive  AllPortsSameDT=off  OutDataTypeStr=boolean
  OR1 : Logic  Operator=OR  IconShape=distinctive  AllPortsSameDT=off  OutDataTypeStr=boolean
  Sum : Outport
  Carry : Outport  Port=2
  wires:
  A/1 -> AND2/1, NOT/1
  B/1 -> OR1/2, NOT1/1
  NOT/1 -> AND/1
  NOT1/1 -> AND1/2, AND/2
  Cin/1 -> AND2/2, NOT2/1
  NOT2/1 -> AND1/1
  AND/1 -> OR/1
  AND1/1 -> OR/2
  OR/1 -> Sum/1
  AND2/1 -> OR1/1
  OR1/1 -> Carry/1

== system Approx_Multiplier_M3_AMA3/AMA3_19 ==
  A : Inport
  B : Inport  Port=2
  Cin : Inport  Port=3
  AND : Logic  IconShape=distinctive  AllPortsSameDT=off  OutDataTypeStr=boolean
  AND1 : Logic  IconShape=distinctive  AllPortsSameDT=off  OutDataTypeStr=boolean
  AND2 : Logic  IconShape=distinctive  AllPortsSameDT=off  OutDataTypeStr=boolean
  NOT : Logic  Operator=NOT  IconShape=distinctive  AllPortsSameDT=off  OutDataTypeStr=boolean
  NOT1 : Logic  Operator=NOT  IconShape=distinctive  AllPortsSameDT=off  OutDataTypeStr=boolean
  NOT2 : Logic  Operator=NOT  IconShape=distinctive  AllPortsSameDT=off  OutDataTypeStr=boolean
  OR : Logic  Operator=OR  IconShape=distinctive  AllPortsSameDT=off  OutDataTypeStr=boolean
  OR1 : Logic  Operator=OR  IconShape=distinctive  AllPortsSameDT=off  OutDataTypeStr=boolean
  Sum : Outport
  Carry : Outport  Port=2
  wires:
  A/1 -> AND2/1, NOT/1
  B/1 -> OR1/2, NOT1/1
  NOT/1 -> AND/1
  NOT1/1 -> AND1/2, AND/2
  Cin/1 -> AND2/2, NOT2/1
  NOT2/1 -> AND1/1
  AND/1 -> OR/1
  AND1/1 -> OR/2
  OR/1 -> Sum/1
  AND2/1 -> OR1/1
  OR1/1 -> Carry/1

== system Approx_Multiplier_M3_AMA3/AMA3_2 ==
  A : Inport
  B : Inport  Port=2
  Cin : Inport  Port=3
  AND : Logic  IconShape=distinctive  AllPortsSameDT=off  OutDataTypeStr=boolean
  AND1 : Logic  IconShape=distinctive  AllPortsSameDT=off  OutDataTypeStr=boolean
  AND2 : Logic  IconShape=distinctive  AllPortsSameDT=off  OutDataTypeStr=boolean
  NOT : Logic  Operator=NOT  IconShape=distinctive  AllPortsSameDT=off  OutDataTypeStr=boolean
  NOT1 : Logic  Operator=NOT  IconShape=distinctive  AllPortsSameDT=off  OutDataTypeStr=boolean
  NOT2 : Logic  Operator=NOT  IconShape=distinctive  AllPortsSameDT=off  OutDataTypeStr=boolean
  OR : Logic  Operator=OR  IconShape=distinctive  AllPortsSameDT=off  OutDataTypeStr=boolean
  OR1 : Logic  Operator=OR  IconShape=distinctive  AllPortsSameDT=off  OutDataTypeStr=boolean
  Sum : Outport
  Carry : Outport  Port=2
  wires:
  A/1 -> AND2/1, NOT/1
  B/1 -> OR1/2, NOT1/1
  NOT/1 -> AND/1
  NOT1/1 -> AND1/2, AND/2
  Cin/1 -> AND2/2, NOT2/1
  NOT2/1 -> AND1/1
  AND/1 -> OR/1
  AND1/1 -> OR/2
  OR/1 -> Sum/1
  AND2/1 -> OR1/1
  OR1/1 -> Carry/1

== system Approx_Multiplier_M3_AMA3/AMA3_20 ==
  A : Inport
  B : Inport  Port=2
  Cin : Inport  Port=3
  AND : Logic  IconShape=distinctive  AllPortsSameDT=off  OutDataTypeStr=boolean
  AND1 : Logic  IconShape=distinctive  AllPortsSameDT=off  OutDataTypeStr=boolean
  AND2 : Logic  IconShape=distinctive  AllPortsSameDT=off  OutDataTypeStr=boolean
  NOT : Logic  Operator=NOT  IconShape=distinctive  AllPortsSameDT=off  OutDataTypeStr=boolean
  NOT1 : Logic  Operator=NOT  IconShape=distinctive  AllPortsSameDT=off  OutDataTypeStr=boolean
  NOT2 : Logic  Operator=NOT  IconShape=distinctive  AllPortsSameDT=off  OutDataTypeStr=boolean
  OR : Logic  Operator=OR  IconShape=distinctive  AllPortsSameDT=off  OutDataTypeStr=boolean
  OR1 : Logic  Operator=OR  IconShape=distinctive  AllPortsSameDT=off  OutDataTypeStr=boolean
  Sum : Outport
  Carry : Outport  Port=2
  wires:
  A/1 -> AND2/1, NOT/1
  B/1 -> OR1/2, NOT1/1
  NOT/1 -> AND/1
  NOT1/1 -> AND1/2, AND/2
  Cin/1 -> AND2/2, NOT2/1
  NOT2/1 -> AND1/1
  AND/1 -> OR/1
  AND1/1 -> OR/2
  OR/1 -> Sum/1
  AND2/1 -> OR1/1
  OR1/1 -> Carry/1

== system Approx_Multiplier_M3_AMA3/AMA3_21 ==
  A : Inport
  B : Inport  Port=2
  Cin : Inport  Port=3
  AND : Logic  IconShape=distinctive  AllPortsSameDT=off  OutDataTypeStr=boolean
  AND1 : Logic  IconShape=distinctive  AllPortsSameDT=off  OutDataTypeStr=boolean
  AND2 : Logic  IconShape=distinctive  AllPortsSameDT=off  OutDataTypeStr=boolean
  NOT : Logic  Operator=NOT  IconShape=distinctive  AllPortsSameDT=off  OutDataTypeStr=boolean
  NOT1 : Logic  Operator=NOT  IconShape=distinctive  AllPortsSameDT=off  OutDataTypeStr=boolean
  NOT2 : Logic  Operator=NOT  IconShape=distinctive  AllPortsSameDT=off  OutDataTypeStr=boolean
  OR : Logic  Operator=OR  IconShape=distinctive  AllPortsSameDT=off  OutDataTypeStr=boolean
  OR1 : Logic  Operator=OR  IconShape=distinctive  AllPortsSameDT=off  OutDataTypeStr=boolean
  Sum : Outport
  Carry : Outport  Port=2
  wires:
  A/1 -> AND2/1, NOT/1
  B/1 -> OR1/2, NOT1/1
  NOT/1 -> AND/1
  NOT1/1 -> AND1/2, AND/2
  Cin/1 -> AND2/2, NOT2/1
  NOT2/1 -> AND1/1
  AND/1 -> OR/1
  AND1/1 -> OR/2
  OR/1 -> Sum/1
  AND2/1 -> OR1/1
  OR1/1 -> Carry/1

== system Approx_Multiplier_M3_AMA3/AMA3_22 ==
  A : Inport
  B : Inport  Port=2
  Cin : Inport  Port=3
  AND : Logic  IconShape=distinctive  AllPortsSameDT=off  OutDataTypeStr=boolean
  AND1 : Logic  IconShape=distinctive  AllPortsSameDT=off  OutDataTypeStr=boolean
  AND2 : Logic  IconShape=distinctive  AllPortsSameDT=off  OutDataTypeStr=boolean
  NOT : Logic  Operator=NOT  IconShape=distinctive  AllPortsSameDT=off  OutDataTypeStr=boolean
  NOT1 : Logic  Operator=NOT  IconShape=distinctive  AllPortsSameDT=off  OutDataTypeStr=boolean
  NOT2 : Logic  Operator=NOT  IconShape=distinctive  AllPortsSameDT=off  OutDataTypeStr=boolean
  OR : Logic  Operator=OR  IconShape=distinctive  AllPortsSameDT=off  OutDataTypeStr=boolean
  OR1 : Logic  Operator=OR  IconShape=distinctive  AllPortsSameDT=off  OutDataTypeStr=boolean
  Sum : Outport
  Carry : Outport  Port=2
  wires:
  A/1 -> AND2/1, NOT/1
  B/1 -> OR1/2, NOT1/1
  NOT/1 -> AND/1
  NOT1/1 -> AND1/2, AND/2
  Cin/1 -> AND2/2, NOT2/1
  NOT2/1 -> AND1/1
  AND/1 -> OR/1
  AND1/1 -> OR/2
  OR/1 -> Sum/1
  AND2/1 -> OR1/1
  OR1/1 -> Carry/1

== system Approx_Multiplier_M3_AMA3/AMA3_23 ==
  A : Inport
  B : Inport  Port=2
  Cin : Inport  Port=3
  AND : Logic  IconShape=distinctive  AllPortsSameDT=off  OutDataTypeStr=boolean
  AND1 : Logic  IconShape=distinctive  AllPortsSameDT=off  OutDataTypeStr=boolean
  AND2 : Logic  IconShape=distinctive  AllPortsSameDT=off  OutDataTypeStr=boolean
  NOT : Logic  Operator=NOT  IconShape=distinctive  AllPortsSameDT=off  OutDataTypeStr=boolean
  NOT1 : Logic  Operator=NOT  IconShape=distinctive  AllPortsSameDT=off  OutDataTypeStr=boolean
  NOT2 : Logic  Operator=NOT  IconShape=distinctive  AllPortsSameDT=off  OutDataTypeStr=boolean
  OR : Logic  Operator=OR  IconShape=distinctive  AllPortsSameDT=off  OutDataTypeStr=boolean
  OR1 : Logic  Operator=OR  IconShape=distinctive  AllPortsSameDT=off  OutDataTypeStr=boolean
  Sum : Outport
  Carry : Outport  Port=2
  wires:
  A/1 -> AND2/1, NOT/1
  B/1 -> OR1/2, NOT1/1
  NOT/1 -> AND/1
  NOT1/1 -> AND1/2, AND/2
  Cin/1 -> AND2/2, NOT2/1
  NOT2/1 -> AND1/1
  AND/1 -> OR/1
  AND1/1 -> OR/2
  OR/1 -> Sum/1
  AND2/1 -> OR1/1
  OR1/1 -> Carry/1

== system Approx_Multiplier_M3_AMA3/AMA3_24 ==
  A : Inport
  B : Inport  Port=2
  Cin : Inport  Port=3
  AND : Logic  IconShape=distinctive  AllPortsSameDT=off  OutDataTypeStr=boolean
  AND1 : Logic  IconShape=distinctive  AllPortsSameDT=off  OutDataTypeStr=boolean
  AND2 : Logic  IconShape=distinctive  AllPortsSameDT=off  OutDataTypeStr=boolean
  NOT : Logic  Operator=NOT  IconShape=distinctive  AllPortsSameDT=off  OutDataTypeStr=boolean
  NOT1 : Logic  Operator=NOT  IconShape=distinctive  AllPortsSameDT=off  OutDataTypeStr=boolean
  NOT2 : Logic  Operator=NOT  IconShape=distinctive  AllPortsSameDT=off  OutDataTypeStr=boolean
  OR : Logic  Operator=OR  IconShape=distinctive  AllPortsSameDT=off  OutDataTypeStr=boolean
  OR1 : Logic  Operator=OR  IconShape=distinctive  AllPortsSameDT=off  OutDataTypeStr=boolean
  Sum : Outport
  Carry : Outport  Port=2
  wires:
  A/1 -> AND2/1, NOT/1
  B/1 -> OR1/2, NOT1/1
  NOT/1 -> AND/1
  NOT1/1 -> AND1/2, AND/2
  Cin/1 -> AND2/2, NOT2/1
  NOT2/1 -> AND1/1
  AND/1 -> OR/1
  AND1/1 -> OR/2
  OR/1 -> Sum/1
  AND2/1 -> OR1/1
  OR1/1 -> Carry/1

== system Approx_Multiplier_M3_AMA3/AMA3_25 ==
  A : Inport
  B : Inport  Port=2
  Cin : Inport  Port=3
  AND : Logic  IconShape=distinctive  AllPortsSameDT=off  OutDataTypeStr=boolean
  AND1 : Logic  IconShape=distinctive  AllPortsSameDT=off  OutDataTypeStr=boolean
  AND2 : Logic  IconShape=distinctive  AllPortsSameDT=off  OutDataTypeStr=boolean
  NOT : Logic  Operator=NOT  IconShape=distinctive  AllPortsSameDT=off  OutDataTypeStr=boolean
  NOT1 : Logic  Operator=NOT  IconShape=distinctive  AllPortsSameDT=off  OutDataTypeStr=boolean
  NOT2 : Logic  Operator=NOT  IconShape=distinctive  AllPortsSameDT=off  OutDataTypeStr=boolean
  OR : Logic  Operator=OR  IconShape=distinctive  AllPortsSameDT=off  OutDataTypeStr=boolean
  OR1 : Logic  Operator=OR  IconShape=distinctive  AllPortsSameDT=off  OutDataTypeStr=boolean
  Sum : Outport
  Carry : Outport  Port=2
  wires:
  A/1 -> AND2/1, NOT/1
  B/1 -> OR1/2, NOT1/1
  NOT/1 -> AND/1
  NOT1/1 -> AND1/2, AND/2
  Cin/1 -> AND2/2, NOT2/1
  NOT2/1 -> AND1/1
  AND/1 -> OR/1
  AND1/1 -> OR/2
  OR/1 -> Sum/1
  AND2/1 -> OR1/1
  OR1/1 -> Carry/1

== system Approx_Multiplier_M3_AMA3/AMA3_26 ==
  A : Inport
  B : Inport  Port=2
  Cin : Inport  Port=3
  AND : Logic  IconShape=distinctive  AllPortsSameDT=off  OutDataTypeStr=boolean
  AND1 : Logic  IconShape=distinctive  AllPortsSameDT=off  OutDataTypeStr=boolean
  AND2 : Logic  IconShape=distinctive  AllPortsSameDT=off  OutDataTypeStr=boolean
  NOT : Logic  Operator=NOT  IconShape=distinctive  AllPortsSameDT=off  OutDataTypeStr=boolean
  NOT1 : Logic  Operator=NOT  IconShape=distinctive  AllPortsSameDT=off  OutDataTypeStr=boolean
  NOT2 : Logic  Operator=NOT  IconShape=distinctive  AllPortsSameDT=off  OutDataTypeStr=boolean
  OR : Logic  Operator=OR  IconShape=distinctive  AllPortsSameDT=off  OutDataTypeStr=boolean
  OR1 : Logic  Operator=OR  IconShape=distinctive  AllPortsSameDT=off  OutDataTypeStr=boolean
  Sum : Outport
  Carry : Outport  Port=2
  wires:
  A/1 -> AND2/1, NOT/1
  B/1 -> OR1/2, NOT1/1
  NOT/1 -> AND/1
  NOT1/1 -> AND1/2, AND/2
  Cin/1 -> AND2/2, NOT2/1
  NOT2/1 -> AND1/1
  AND/1 -> OR/1
  AND1/1 -> OR/2
  OR/1 -> Sum/1
  AND2/1 -> OR1/1
  OR1/1 -> Carry/1

== system Approx_Multiplier_M3_AMA3/AMA3_27 ==
  A : Inport
  B : Inport  Port=2
  Cin : Inport  Port=3
  AND : Logic  IconShape=distinctive  AllPortsSameDT=off  OutDataTypeStr=boolean
  AND1 : Logic  IconShape=distinctive  AllPortsSameDT=off  OutDataTypeStr=boolean
  AND2 : Logic  IconShape=distinctive  AllPortsSameDT=off  OutDataTypeStr=boolean
  NOT : Logic  Operator=NOT  IconShape=distinctive  AllPortsSameDT=off  OutDataTypeStr=boolean
  NOT1 : Logic  Operator=NOT  IconShape=distinctive  AllPortsSameDT=off  OutDataTypeStr=boolean
  NOT2 : Logic  Operator=NOT  IconShape=distinctive  AllPortsSameDT=off  OutDataTypeStr=boolean
  OR : Logic  Operator=OR  IconShape=distinctive  AllPortsSameDT=off  OutDataTypeStr=boolean
  OR1 : Logic  Operator=OR  IconShape=distinctive  AllPortsSameDT=off  OutDataTypeStr=boolean
  Sum : Outport
  Carry : Outport  Port=2
  wires:
  A/1 -> AND2/1, NOT/1
  B/1 -> OR1/2, NOT1/1
  NOT/1 -> AND/1
  NOT1/1 -> AND1/2, AND/2
  Cin/1 -> AND2/2, NOT2/1
  NOT2/1 -> AND1/1
  AND/1 -> OR/1
  AND1/1 -> OR/2
  OR/1 -> Sum/1
  AND2/1 -> OR1/1
  OR1/1 -> Carry/1

== system Approx_Multiplier_M3_AMA3/AMA3_28 ==
  A : Inport
  B : Inport  Port=2
  Cin : Inport  Port=3
  AND : Logic  IconShape=distinctive  AllPortsSameDT=off  OutDataTypeStr=boolean
  AND1 : Logic  IconShape=distinctive  AllPortsSameDT=off  OutDataTypeStr=boolean
  AND2 : Logic  IconShape=distinctive  AllPortsSameDT=off  OutDataTypeStr=boolean
  NOT : Logic  Operator=NOT  IconShape=distinctive  AllPortsSameDT=off  OutDataTypeStr=boolean
  NOT1 : Logic  Operator=NOT  IconShape=distinctive  AllPortsSameDT=off  OutDataTypeStr=boolean
  NOT2 : Logic  Operator=NOT  IconShape=distinctive  AllPortsSameDT=off  OutDataTypeStr=boolean
  OR : Logic  Operator=OR  IconShape=distinctive  AllPortsSameDT=off  OutDataTypeStr=boolean
  OR1 : Logic  Operator=OR  IconShape=distinctive  AllPortsSameDT=off  OutDataTypeStr=boolean
  Sum : Outport
  Carry : Outport  Port=2
  wires:
  A/1 -> AND2/1, NOT/1
  B/1 -> OR1/2, NOT1/1
  NOT/1 -> AND/1
  NOT1/1 -> AND1/2, AND/2
  Cin/1 -> AND2/2, NOT2/1
  NOT2/1 -> AND1/1
  AND/1 -> OR/1
  AND1/1 -> OR/2
  OR/1 -> Sum/1
  AND2/1 -> OR1/1
  OR1/1 -> Carry/1

== system Approx_Multiplier_M3_AMA3/AMA3_3 ==
  A : Inport
  B : Inport  Port=2
  Cin : Inport  Port=3
  AND : Logic  IconShape=distinctive  AllPortsSameDT=off  OutDataTypeStr=boolean
  AND1 : Logic  IconShape=distinctive  AllPortsSameDT=off  OutDataTypeStr=boolean
  AND2 : Logic  IconShape=distinctive  AllPortsSameDT=off  OutDataTypeStr=boolean
  NOT : Logic  Operator=NOT  IconShape=distinctive  AllPortsSameDT=off  OutDataTypeStr=boolean
  NOT1 : Logic  Operator=NOT  IconShape=distinctive  AllPortsSameDT=off  OutDataTypeStr=boolean
  NOT2 : Logic  Operator=NOT  IconShape=distinctive  AllPortsSameDT=off  OutDataTypeStr=boolean
  OR : Logic  Operator=OR  IconShape=distinctive  AllPortsSameDT=off  OutDataTypeStr=boolean
  OR1 : Logic  Operator=OR  IconShape=distinctive  AllPortsSameDT=off  OutDataTypeStr=boolean
  Sum : Outport
  Carry : Outport  Port=2
  wires:
  A/1 -> AND2/1, NOT/1
  B/1 -> OR1/2, NOT1/1
  NOT/1 -> AND/1
  NOT1/1 -> AND1/2, AND/2
  Cin/1 -> AND2/2, NOT2/1
  NOT2/1 -> AND1/1
  AND/1 -> OR/1
  AND1/1 -> OR/2
  OR/1 -> Sum/1
  AND2/1 -> OR1/1
  OR1/1 -> Carry/1

== system Approx_Multiplier_M3_AMA3/AMA3_4 ==
  A : Inport
  B : Inport  Port=2
  Cin : Inport  Port=3
  AND : Logic  IconShape=distinctive  AllPortsSameDT=off  OutDataTypeStr=boolean
  AND1 : Logic  IconShape=distinctive  AllPortsSameDT=off  OutDataTypeStr=boolean
  AND2 : Logic  IconShape=distinctive  AllPortsSameDT=off  OutDataTypeStr=boolean
  NOT : Logic  Operator=NOT  IconShape=distinctive  AllPortsSameDT=off  OutDataTypeStr=boolean
  NOT1 : Logic  Operator=NOT  IconShape=distinctive  AllPortsSameDT=off  OutDataTypeStr=boolean
  NOT2 : Logic  Operator=NOT  IconShape=distinctive  AllPortsSameDT=off  OutDataTypeStr=boolean
  OR : Logic  Operator=OR  IconShape=distinctive  AllPortsSameDT=off  OutDataTypeStr=boolean
  OR1 : Logic  Operator=OR  IconShape=distinctive  AllPortsSameDT=off  OutDataTypeStr=boolean
  Sum : Outport
  Carry : Outport  Port=2
  wires:
  A/1 -> AND2/1, NOT/1
  B/1 -> OR1/2, NOT1/1
  NOT/1 -> AND/1
  NOT1/1 -> AND1/2, AND/2
  Cin/1 -> AND2/2, NOT2/1
  NOT2/1 -> AND1/1
  AND/1 -> OR/1
  AND1/1 -> OR/2
  OR/1 -> Sum/1
  AND2/1 -> OR1/1
  OR1/1 -> Carry/1

== system Approx_Multiplier_M3_AMA3/AMA3_5 ==
  A : Inport
  B : Inport  Port=2
  Cin : Inport  Port=3
  AND : Logic  IconShape=distinctive  AllPortsSameDT=off  OutDataTypeStr=boolean
  AND1 : Logic  IconShape=distinctive  AllPortsSameDT=off  OutDataTypeStr=boolean
  AND2 : Logic  IconShape=distinctive  AllPortsSameDT=off  OutDataTypeStr=boolean
  NOT : Logic  Operator=NOT  IconShape=distinctive  AllPortsSameDT=off  OutDataTypeStr=boolean
  NOT1 : Logic  Operator=NOT  IconShape=distinctive  AllPortsSameDT=off  OutDataTypeStr=boolean
  NOT2 : Logic  Operator=NOT  IconShape=distinctive  AllPortsSameDT=off  OutDataTypeStr=boolean
  OR : Logic  Operator=OR  IconShape=distinctive  AllPortsSameDT=off  OutDataTypeStr=boolean
  OR1 : Logic  Operator=OR  IconShape=distinctive  AllPortsSameDT=off  OutDataTypeStr=boolean
  Sum : Outport
  Carry : Outport  Port=2
  wires:
  A/1 -> AND2/1, NOT/1
  B/1 -> OR1/2, NOT1/1
  NOT/1 -> AND/1
  NOT1/1 -> AND1/2, AND/2
  Cin/1 -> AND2/2, NOT2/1
  NOT2/1 -> AND1/1
  AND/1 -> OR/1
  AND1/1 -> OR/2
  OR/1 -> Sum/1
  AND2/1 -> OR1/1
  OR1/1 -> Carry/1

== system Approx_Multiplier_M3_AMA3/AMA3_6 ==
  A : Inport
  B : Inport  Port=2
  Cin : Inport  Port=3
  AND : Logic  IconShape=distinctive  AllPortsSameDT=off  OutDataTypeStr=boolean
  AND1 : Logic  IconShape=distinctive  AllPortsSameDT=off  OutDataTypeStr=boolean
  AND2 : Logic  IconShape=distinctive  AllPortsSameDT=off  OutDataTypeStr=boolean
  NOT : Logic  Operator=NOT  IconShape=distinctive  AllPortsSameDT=off  OutDataTypeStr=boolean
  NOT1 : Logic  Operator=NOT  IconShape=distinctive  AllPortsSameDT=off  OutDataTypeStr=boolean
  NOT2 : Logic  Operator=NOT  IconShape=distinctive  AllPortsSameDT=off  OutDataTypeStr=boolean
  OR : Logic  Operator=OR  IconShape=distinctive  AllPortsSameDT=off  OutDataTypeStr=boolean
  OR1 : Logic  Operator=OR  IconShape=distinctive  AllPortsSameDT=off  OutDataTypeStr=boolean
  Sum : Outport
  Carry : Outport  Port=2
  wires:
  A/1 -> AND2/1, NOT/1
  B/1 -> OR1/2, NOT1/1
  NOT/1 -> AND/1
  NOT1/1 -> AND1/2, AND/2
  Cin/1 -> AND2/2, NOT2/1
  NOT2/1 -> AND1/1
  AND/1 -> OR/1
  AND1/1 -> OR/2
  OR/1 -> Sum/1
  AND2/1 -> OR1/1
  OR1/1 -> Carry/1

== system Approx_Multiplier_M3_AMA3/AMA3_7 ==
  A : Inport
  B : Inport  Port=2
  Cin : Inport  Port=3
  AND : Logic  IconShape=distinctive  AllPortsSameDT=off  OutDataTypeStr=boolean
  AND1 : Logic  IconShape=distinctive  AllPortsSameDT=off  OutDataTypeStr=boolean
  AND2 : Logic  IconShape=distinctive  AllPortsSameDT=off  OutDataTypeStr=boolean
  NOT : Logic  Operator=NOT  IconShape=distinctive  AllPortsSameDT=off  OutDataTypeStr=boolean
  NOT1 : Logic  Operator=NOT  IconShape=distinctive  AllPortsSameDT=off  OutDataTypeStr=boolean
  NOT2 : Logic  Operator=NOT  IconShape=distinctive  AllPortsSameDT=off  OutDataTypeStr=boolean
  OR : Logic  Operator=OR  IconShape=distinctive  AllPortsSameDT=off  OutDataTypeStr=boolean
  OR1 : Logic  Operator=OR  IconShape=distinctive  AllPortsSameDT=off  OutDataTypeStr=boolean
  Sum : Outport
  Carry : Outport  Port=2
  wires:
  A/1 -> AND2/1, NOT/1
  B/1 -> OR1/2, NOT1/1
  NOT/1 -> AND/1
  NOT1/1 -> AND1/2, AND/2
  Cin/1 -> AND2/2, NOT2/1
  NOT2/1 -> AND1/1
  AND/1 -> OR/1
  AND1/1 -> OR/2
  OR/1 -> Sum/1
  AND2/1 -> OR1/1
  OR1/1 -> Carry/1

== system Approx_Multiplier_M3_AMA3/AMA3_8 ==
  A : Inport
  B : Inport  Port=2
  Cin : Inport  Port=3
  AND : Logic  IconShape=distinctive  AllPortsSameDT=off  OutDataTypeStr=boolean
  AND1 : Logic  IconShape=distinctive  AllPortsSameDT=off  OutDataTypeStr=boolean
  AND2 : Logic  IconShape=distinctive  AllPortsSameDT=off  OutDataTypeStr=boolean
  NOT : Logic  Operator=NOT  IconShape=distinctive  AllPortsSameDT=off  OutDataTypeStr=boolean
  NOT1 : Logic  Operator=NOT  IconShape=distinctive  AllPortsSameDT=off  OutDataTypeStr=boolean
  NOT2 : Logic  Operator=NOT  IconShape=distinctive  AllPortsSameDT=off  OutDataTypeStr=boolean
  OR : Logic  Operator=OR  IconShape=distinctive  AllPortsSameDT=off  OutDataTypeStr=boolean
  OR1 : Logic  Operator=OR  IconShape=distinctive  AllPortsSameDT=off  OutDataTypeStr=boolean
  Sum : Outport
  Carry : Outport  Port=2
  wires:
  A/1 -> AND2/1, NOT/1
  B/1 -> OR1/2, NOT1/1
  NOT/1 -> AND/1
  NOT1/1 -> AND1/2, AND/2
  Cin/1 -> AND2/2, NOT2/1
  NOT2/1 -> AND1/1
  AND/1 -> OR/1
  AND1/1 -> OR/2
  OR/1 -> Sum/1
  AND2/1 -> OR1/1
  OR1/1 -> Carry/1

== system Approx_Multiplier_M3_AMA3/AMA3_9 ==
  A : Inport
  B : Inport  Port=2
  Cin : Inport  Port=3
  AND : Logic  IconShape=distinctive  AllPortsSameDT=off  OutDataTypeStr=boolean
  AND1 : Logic  IconShape=distinctive  AllPortsSameDT=off  OutDataTypeStr=boolean
  AND2 : Logic  IconShape=distinctive  AllPortsSameDT=off  OutDataTypeStr=boolean
  NOT : Logic  Operator=NOT  IconShape=distinctive  AllPortsSameDT=off  OutDataTypeStr=boolean
  NOT1 : Logic  Operator=NOT  IconShape=distinctive  AllPortsSameDT=off  OutDataTypeStr=boolean
  NOT2 : Logic  Operator=NOT  IconShape=distinctive  AllPortsSameDT=off  OutDataTypeStr=boolean
  OR : Logic  Operator=OR  IconShape=distinctive  AllPortsSameDT=off  OutDataTypeStr=boolean
  OR1 : Logic  Operator=OR  IconShape=distinctive  AllPortsSameDT=off  OutDataTypeStr=boolean
  Sum : Outport
  Carry : Outport  Port=2
  wires:
  A/1 -> AND2/1, NOT/1
  B/1 -> OR1/2, NOT1/1
  NOT/1 -> AND/1
  NOT1/1 -> AND1/2, AND/2
  Cin/1 -> AND2/2, NOT2/1
  NOT2/1 -> AND1/1
  AND/1 -> OR/1
  AND1/1 -> OR/2
  OR/1 -> Sum/1
  AND2/1 -> OR1/1
  OR1/1 -> Carry/1

== system Approx_Multiplier_M3_AMA3/Full Adder12 ==
  A : Inport
  B : Inport  Port=2
  Cin : Inport  Port=3
  Half Adder : Subsystem
  Half Adder1 : Subsystem
  Logical Operator : Logic  Operator=OR  AllPortsSameDT=off  OutDataTypeStr=boolean
  Sum : Outport
  Carry : Outport  Port=2
  wires:
  Cin/1 -> Half Adder1/1(In)
  Half Adder1/2(Cout) -> Logical Operator/1
  Half Adder/1(Sum) -> Half Adder1/2(Cin)
  Half Adder1/1(Sum) -> Sum/1
  Half Adder/2(Cout) -> Logical Operator/2
  A/1 -> Half Adder/1(In)
  B/1 -> Half Adder/2(Cin)
  Logical Operator/1 -> Carry/1
